simulink model "Moteur"  (R2018a)
settings: Solver=ode15s  StartTime=0.0  StopTime=10.0  FixedStep=0.0001  RelTol=1e-3
libraries: cstblocks x1
settings Model: Creator=chsira  LastModifiedBy=charl
settings DataIOCC: SaveOutput=off  SaveTime=off
settings DebuggingCC: LibraryContextMissingDiagnostic=warning
settings SFSimCC: SimUseLocalCustomCode=on
settings RTWCC: RTWUseLocalCustomCode=on

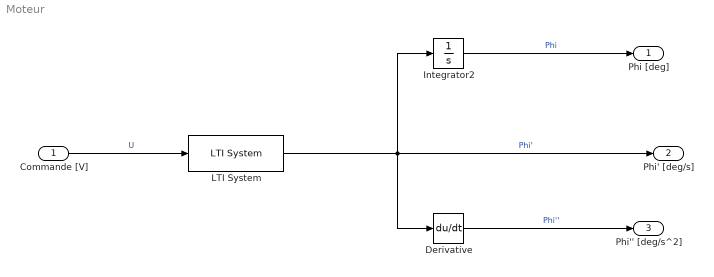
== system Moteur ==
  Commande [V] : Inport  OutDataTypeStr=double  PortDimensions=1  SampleTime=0
  Derivative : Derivative
  Integrator2 : Integrator
  LTI System : cstblocks/LTI System  sys=H  IC=[]
  Phi [deg] : Outport  OutDataTypeStr=double  PortDimensions=1  SampleTime=0
  Phi' [deg/s] : Outport  Port=2  OutDataTypeStr=double  PortDimensions=1  SampleTime=0
  "Phi'' [deg/s^2] " : Outport  Port=3  OutDataTypeStr=double  PortDimensions=1  SampleTime=0
  wires:
  Commande [V]/1 -> LTI System/1  "U"
  LTI System/1 -> Phi' [deg/s]/1, Integrator2/1, Derivative/1  "Phi'"
  Integrator2/1 -> Phi [deg]/1  "Phi"
  Derivative/1 -> "Phi'' [deg/s^2] "/1  "Phi''"
